simulink model "hydraulicsystem"  (R2020b)
settings: Solver=VariableStepAuto  StartTime=0.0  StopTime=80  FixedStep=0.01  RelTol=1e-3
libraries: fl_lib x15, sh_lib x7, nesl_utility x6, simulink x3, dspstat3 x1, sdl_lib x1
settings Model: EnablePacing=on  PacingRate=2  Creator=mateu  LastModifiedBy=mateu
settings SolverCC: ZeroCrossControl=EnableAll  ZeroCrossAlgorithm=Adaptive  AlgebraicLoopSolver=LineSearch
settings DebuggingCC: IgnoredZcDiagnostic=none
settings SimscapeCC: GlobalZcOffDiagnosticOptions=error  SimscapeLogOpenViewer=on  SimscapeLogLimitData=off

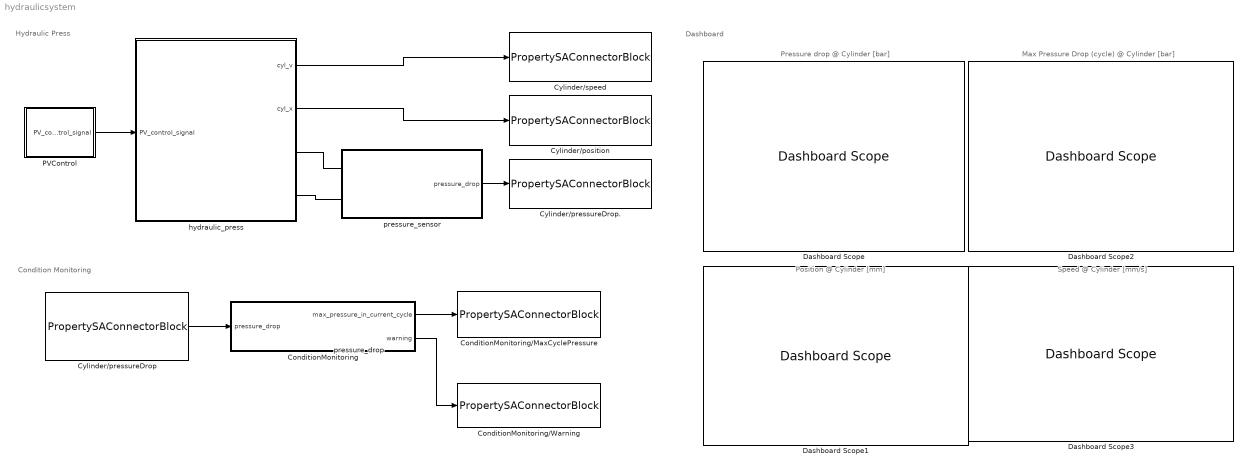
== system hydraulicsystem ==
  note: Dashboard
  note: Hydraulic Press
  note: Condition Monitoring
  note: Pressure drop @ Cylinder [bar]
  note: Max Pressure Drop (cycle) @ Cylinder [bar]
  note: Position @ Cylinder [mm]
  note: Speed @ Cylinder [mm/s]
  pressure_drop : Inport
  ConditionMonitoring : Subsystem
  ConditionMonitoring/MaxCyclePressure : S-Function  FunctionName=PropertySAConnectorBlock  Parameters=bm, sr, regUrlStr, aasUrlStr, aasId, smId, seId  SFunctionDeploymentMode=off  EnableBusSupport=off  mask{bmStr=Real-time, conMethod=via RegistryServer, aasUrlStr_=http://localhost:4001/aasServer/shells/https%3A%2F%2Fexample.com%2Fids%2Faas%2F6001_2130_8022_6165/aas, regUrlStr=http://localhost:8082/registry/api/v1/registry, sr=0.1, aasId=HydraulicPress, smId=ConditionMonitoring, seId=maxCyclePressure, bm=1, aasUrlStr=}
      mask prompts: bmStr "Operation Mode"; conMethod "Connection Method"; aasUrlStr_ "AAS Url"; regUrlStr "Registry URL"; sr "Sample Rate"; aasId "AAS Id"; smId "Submodel IdShort"; seId "Property IdShort"
      mask TypeOptions bmStr: Snapshot | Real-time
      mask Callback bmStr:
      | bmStr = get_param(gcb,'bmStr');
      | vis = get_param(gcb,'MaskVisibilities');
      | 
      | switch bmStr
      |     case 'Snapshot'
      |         set_param(gcb, 'bm', "0");
      |         vis(5) = {'off'};
      |         set_param(gcb, 'MaskVisibilities', vis);
      |     case 'Real-time'
      |         set_param(gcb, 'bm',  "1");
      |         vis(5) = {'on'};
      |         set_param(gcb, 'MaskVisibilities', vis);
      | end
      mask TypeOptions conMethod: via RegistryServer | via AAS URL
      mask Callback conMethod:
      | conMethod = get_param(gcb,'conMethod');
      | aasUrlStr = get_param(gcb,'aasUrlStr_');
      | vis = get_param(gcb,'MaskVisibilities');
      | 
      | switch conMethod
      |     case 'via RegistryServer'
      |         vis(3) = {'off'};
      |         vis(4) = {'on'};
      |         set_param(gcb, 'MaskVisibilities', vis);
      |         set_param(gcb, 'aasUrlStr', '');
      |     case 'via AAS URL'
      |         vis(3) = {'on'};
      |         vis(4) = {'off'};
      |         set_param(gcb, 'MaskVisibilities', vis);
      |         set_param(gcb, 'aasUrlStr', aasUrlStr);
      | end
      mask Callback aasUrlStr_:
      | conMethod = get_param(gcb,'conMethod');
      | aasUrlStr = get_param(gcb,'aasUrlStr_');
      | switch conMethod
      |     case 'via AAS URL'
      |         set_param(gcb, 'aasUrlStr', aasUrlStr);
      | end
      mask DialogControl DescGroupVar Prompt: Standalone Property Block
      mask DialogControl DescTextVar Prompt: This block connects to a SubmodelElement running in an AAS Server. Data sent to the block's input updates the value of the SubmodelElement, whereas its current value is sent to the block's output. This process can be executed in two operation modes: Snapshot mode, wherein the input routine is executed at the beginining and the output routine at the end of the simulation; Real-time mode, by which is assumed that the wall clock is the same as the simulation clock and the input/output routines are executed in the specified sample rate.
      mask Display:
      | bm = get_param(gcb,'bm')
      | sr = get_param(gcb,'sr')
      | aas = replace(get_param(gcb,'aasId'),"_","\_");
      | sm = replace(get_param(gcb,'smId'),"_","\_");
      | se = replace(get_param(gcb,'seId'),"_","\_");
      | 
      | pos = get_param(gcb, 'Position');
      | w = pos(3) - pos(1);
      | h = pos(4) - pos(2);
      | 
      | full = sm  + "/" + se
      | text(5,20, "{\bf\fontsize{7}"+aas+"}", 'texmode','on')
      | text(5,10, "{\bf\fontsize{6}"+full+"}", 'texmode','on')
      | image('basyx.png', [w-15,h-20,10,15]);
      | 
      | if bm=="1"
      |     port_label('output', 1,"{\bf\fontsize{6}sr="+sr+"s}", 'texmode','on')
      | end
  ConditionMonitoring/Warning : S-Function  FunctionName=PropertySAConnectorBlock  Parameters=bm, sr, regUrlStr, aasUrlStr, aasId, smId, seId  SFunctionDeploymentMode=off  EnableBusSupport=off  mask{bmStr=Real-time, conMethod=via RegistryServer, aasUrlStr_=http://localhost:4001/aasServer/shells/https%3A%2F%2Fexample.com%2Fids%2Faas%2F6001_2130_8022_6165/aas, regUrlStr=http://localhost:8082/registry/api/v1/registry, sr=0.1, aasId=HydraulicPress, smId=ConditionMonitoring, seId=warning, bm=1, aasUrlStr=}
      mask prompts: bmStr "Operation Mode"; conMethod "Connection Method"; aasUrlStr_ "AAS Url"; regUrlStr "Registry URL"; sr "Sample Rate"; aasId "AAS Id"; smId "Submodel IdShort"; seId "Property IdShort"
      mask TypeOptions bmStr: Snapshot | Real-time
      mask Callback bmStr:
      | bmStr = get_param(gcb,'bmStr');
      | vis = get_param(gcb,'MaskVisibilities');
      | 
      | switch bmStr
      |     case 'Snapshot'
      |         set_param(gcb, 'bm', "0");
      |         vis(5) = {'off'};
      |         set_param(gcb, 'MaskVisibilities', vis);
      |     case 'Real-time'
      |         set_param(gcb, 'bm',  "1");
      |         vis(5) = {'on'};
      |         set_param(gcb, 'MaskVisibilities', vis);
      | end
      mask TypeOptions conMethod: via RegistryServer | via AAS URL
      mask Callback conMethod:
      | conMethod = get_param(gcb,'conMethod');
      | aasUrlStr = get_param(gcb,'aasUrlStr_');
      | vis = get_param(gcb,'MaskVisibilities');
      | 
      | switch conMethod
      |     case 'via RegistryServer'
      |         vis(3) = {'off'};
      |         vis(4) = {'on'};
      |         set_param(gcb, 'MaskVisibilities', vis);
      |         set_param(gcb, 'aasUrlStr', '');
      |     case 'via AAS URL'
      |         vis(3) = {'on'};
      |         vis(4) = {'off'};
      |         set_param(gcb, 'MaskVisibilities', vis);
      |         set_param(gcb, 'aasUrlStr', aasUrlStr);
      | end
      mask Callback aasUrlStr_:
      | conMethod = get_param(gcb,'conMethod');
      | aasUrlStr = get_param(gcb,'aasUrlStr_');
      | switch conMethod
      |     case 'via AAS URL'
      |         set_param(gcb, 'aasUrlStr', aasUrlStr);
      | end
      mask DialogControl DescGroupVar Prompt: Standalone Property Block
      mask DialogControl DescTextVar Prompt: This block connects to a SubmodelElement running in an AAS Server. Data sent to the block's input updates the value of the SubmodelElement, whereas its current value is sent to the block's output. This process can be executed in two operation modes: Snapshot mode, wherein the input routine is executed at the beginining and the output routine at the end of the simulation; Real-time mode, by which is assumed that the wall clock is the same as the simulation clock and the input/output routines are executed in the specified sample rate.
      mask Display:
      | bm = get_param(gcb,'bm')
      | sr = get_param(gcb,'sr')
      | aas = replace(get_param(gcb,'aasId'),"_","\_");
      | sm = replace(get_param(gcb,'smId'),"_","\_");
      | se = replace(get_param(gcb,'seId'),"_","\_");
      | 
      | pos = get_param(gcb, 'Position');
      | w = pos(3) - pos(1);
      | h = pos(4) - pos(2);
      | 
      | full = sm  + "/" + se
      | text(5,20, "{\bf\fontsize{7}"+aas+"}", 'texmode','on')
      | text(5,10, "{\bf\fontsize{6}"+full+"}", 'texmode','on')
      | image('basyx.png', [w-15,h-20,10,15]);
      | 
      | if bm=="1"
      |     port_label('output', 1,"{\bf\fontsize{6}sr="+sr+"s}", 'texmode','on')
      | end
  Cylinder/position : S-Function  FunctionName=PropertySAConnectorBlock  Parameters=bm, sr, regUrlStr, aasUrlStr, aasId, smId, seId  SFunctionDeploymentMode=off  EnableBusSupport=off  mask{bmStr=Real-time, conMethod=via RegistryServer, aasUrlStr_=http://localhost:4001/aasServer/shells/https%3A%2F%2Fexample.com%2Fids%2Faas%2F6001_2130_8022_6165/aas, regUrlStr=http://localhost:8082/registry/api/v1/registry, sr=0.1, aasId=HydraulicPress, smId=Cylinder, seId=position, bm=1, aasUrlStr=}
      mask prompts: bmStr "Operation Mode"; conMethod "Connection Method"; aasUrlStr_ "AAS Url"; regUrlStr "Registry URL"; sr "Sample Rate"; aasId "AAS Id"; smId "Submodel IdShort"; seId "Property IdShort"
      mask TypeOptions bmStr: Snapshot | Real-time
      mask Callback bmStr:
      | bmStr = get_param(gcb,'bmStr');
      | vis = get_param(gcb,'MaskVisibilities');
      | 
      | switch bmStr
      |     case 'Snapshot'
      |         set_param(gcb, 'bm', "0");
      |         vis(5) = {'off'};
      |         set_param(gcb, 'MaskVisibilities', vis);
      |     case 'Real-time'
      |         set_param(gcb, 'bm',  "1");
      |         vis(5) = {'on'};
      |         set_param(gcb, 'MaskVisibilities', vis);
      | end
      mask TypeOptions conMethod: via RegistryServer | via AAS URL
      mask Callback conMethod:
      | conMethod = get_param(gcb,'conMethod');
      | aasUrlStr = get_param(gcb,'aasUrlStr_');
      | vis = get_param(gcb,'MaskVisibilities');
      | 
      | switch conMethod
      |     case 'via RegistryServer'
      |         vis(3) = {'off'};
      |         vis(4) = {'on'};
      |         set_param(gcb, 'MaskVisibilities', vis);
      |         set_param(gcb, 'aasUrlStr', '');
      |     case 'via AAS URL'
      |         vis(3) = {'on'};
      |         vis(4) = {'off'};
      |         set_param(gcb, 'MaskVisibilities', vis);
      |         set_param(gcb, 'aasUrlStr', aasUrlStr);
      | end
      mask Callback aasUrlStr_:
      | conMethod = get_param(gcb,'conMethod');
      | aasUrlStr = get_param(gcb,'aasUrlStr_');
      | switch conMethod
      |     case 'via AAS URL'
      |         set_param(gcb, 'aasUrlStr', aasUrlStr);
      | end
      mask DialogControl DescGroupVar Prompt: Standalone Property Block
      mask DialogControl DescTextVar Prompt: This block connects to a SubmodelElement running in an AAS Server. Data sent to the block's input updates the value of the SubmodelElement, whereas its current value is sent to the block's output. This process can be executed in two operation modes: Snapshot mode, wherein the input routine is executed at the beginining and the output routine at the end of the simulation; Real-time mode, by which is assumed that the wall clock is the same as the simulation clock and the input/output routines are executed in the specified sample rate.
      mask Display:
      | bm = get_param(gcb,'bm')
      | sr = get_param(gcb,'sr')
      | aas = replace(get_param(gcb,'aasId'),"_","\_");
      | sm = replace(get_param(gcb,'smId'),"_","\_");
      | se = replace(get_param(gcb,'seId'),"_","\_");
      | 
      | pos = get_param(gcb, 'Position');
      | w = pos(3) - pos(1);
      | h = pos(4) - pos(2);
      | 
      | full = sm  + "/" + se
      | text(5,20, "{\bf\fontsize{7}"+aas+"}", 'texmode','on')
      | text(5,10, "{\bf\fontsize{6}"+full+"}", 'texmode','on')
      | image('basyx.png', [w-15,h-20,10,15]);
      | 
      | if bm=="1"
      |     port_label('output', 1,"{\bf\fontsize{6}sr="+sr+"s}", 'texmode','on')
      | end
  Cylinder/pressureDrop : S-Function  FunctionName=PropertySAConnectorBlock  Parameters=bm, sr, regUrlStr, aasUrlStr, aasId, smId, seId  SFunctionDeploymentMode=off  EnableBusSupport=off  mask{bmStr=Real-time, conMethod=via RegistryServer, aasUrlStr_=http://localhost:4001/aasServer/shells/https%3A%2F%2Fexample.com%2Fids%2Faas%2F6001_2130_8022_6165/aas, regUrlStr=http://localhost:8082/registry/api/v1/registry, sr=0.1, aasId=HydraulicPress, smId=Cylinder, seId=pressureDrop, bm=1, aasUrlStr=}
      mask prompts: bmStr "Operation Mode"; conMethod "Connection Method"; aasUrlStr_ "AAS Url"; regUrlStr "Registry URL"; sr "Sample Rate"; aasId "AAS Id"; smId "Submodel IdShort"; seId "Property IdShort"
      mask TypeOptions bmStr: Snapshot | Real-time
      mask Callback bmStr:
      | bmStr = get_param(gcb,'bmStr');
      | vis = get_param(gcb,'MaskVisibilities');
      | 
      | switch bmStr
      |     case 'Snapshot'
      |         set_param(gcb, 'bm', "0");
      |         vis(5) = {'off'};
      |         set_param(gcb, 'MaskVisibilities', vis);
      |     case 'Real-time'
      |         set_param(gcb, 'bm',  "1");
      |         vis(5) = {'on'};
      |         set_param(gcb, 'MaskVisibilities', vis);
      | end
      mask TypeOptions conMethod: via RegistryServer | via AAS URL
      mask Callback conMethod:
      | conMethod = get_param(gcb,'conMethod');
      | aasUrlStr = get_param(gcb,'aasUrlStr_');
      | vis = get_param(gcb,'MaskVisibilities');
      | 
      | switch conMethod
      |     case 'via RegistryServer'
      |         vis(3) = {'off'};
      |         vis(4) = {'on'};
      |         set_param(gcb, 'MaskVisibilities', vis);
      |         set_param(gcb, 'aasUrlStr', '');
      |     case 'via AAS URL'
      |         vis(3) = {'on'};
      |         vis(4) = {'off'};
      |         set_param(gcb, 'MaskVisibilities', vis);
      |         set_param(gcb, 'aasUrlStr', aasUrlStr);
      | end
      mask Callback aasUrlStr_:
      | conMethod = get_param(gcb,'conMethod');
      | aasUrlStr = get_param(gcb,'aasUrlStr_');
      | switch conMethod
      |     case 'via AAS URL'
      |         set_param(gcb, 'aasUrlStr', aasUrlStr);
      | end
      mask DialogControl DescGroupVar Prompt: Standalone Property Block
      mask DialogControl DescTextVar Prompt: This block connects to a SubmodelElement running in an AAS Server. Data sent to the block's input updates the value of the SubmodelElement, whereas its current value is sent to the block's output. This process can be executed in two operation modes: Snapshot mode, wherein the input routine is executed at the beginining and the output routine at the end of the simulation; Real-time mode, by which is assumed that the wall clock is the same as the simulation clock and the input/output routines are executed in the specified sample rate.
      mask Display:
      | bm = get_param(gcb,'bm')
      | sr = get_param(gcb,'sr')
      | aas = replace(get_param(gcb,'aasId'),"_","\_");
      | sm = replace(get_param(gcb,'smId'),"_","\_");
      | se = replace(get_param(gcb,'seId'),"_","\_");
      | 
      | pos = get_param(gcb, 'Position');
      | w = pos(3) - pos(1);
      | h = pos(4) - pos(2);
      | 
      | full = sm  + "/" + se
      | text(5,20, "{\bf\fontsize{7}"+aas+"}", 'texmode','on')
      | text(5,10, "{\bf\fontsize{6}"+full+"}", 'texmode','on')
      | image('basyx.png', [w-15,h-20,10,15]);
      | 
      | if bm=="1"
      |     port_label('output', 1,"{\bf\fontsize{6}sr="+sr+"s}", 'texmode','on')
      | end
  Cylinder/pressureDrop. : S-Function  FunctionName=PropertySAConnectorBlock  Parameters=bm, sr, regUrlStr, aasUrlStr, aasId, smId, seId  SFunctionDeploymentMode=off  EnableBusSupport=off  mask{bmStr=Real-time, conMethod=via RegistryServer, aasUrlStr_=http://localhost:4001/aasServer/shells/https%3A%2F%2Fexample.com%2Fids%2Faas%2F6001_2130_8022_6165/aas, regUrlStr=http://localhost:8082/registry/api/v1/registry, sr=0.05, aasId=HydraulicPress, smId=Cylinder, seId=pressureDrop, bm=1, aasUrlStr=}
      mask prompts: bmStr "Operation Mode"; conMethod "Connection Method"; aasUrlStr_ "AAS Url"; regUrlStr "Registry URL"; sr "Sample Rate"; aasId "AAS Id"; smId "Submodel IdShort"; seId "Property IdShort"
      mask TypeOptions bmStr: Snapshot | Real-time
      mask Callback bmStr:
      | bmStr = get_param(gcb,'bmStr');
      | vis = get_param(gcb,'MaskVisibilities');
      | 
      | switch bmStr
      |     case 'Snapshot'
      |         set_param(gcb, 'bm', "0");
      |         vis(5) = {'off'};
      |         set_param(gcb, 'MaskVisibilities', vis);
      |     case 'Real-time'
      |         set_param(gcb, 'bm',  "1");
      |         vis(5) = {'on'};
      |         set_param(gcb, 'MaskVisibilities', vis);
      | end
      mask TypeOptions conMethod: via RegistryServer | via AAS URL
      mask Callback conMethod:
      | conMethod = get_param(gcb,'conMethod');
      | aasUrlStr = get_param(gcb,'aasUrlStr_');
      | vis = get_param(gcb,'MaskVisibilities');
      | 
      | switch conMethod
      |     case 'via RegistryServer'
      |         vis(3) = {'off'};
      |         vis(4) = {'on'};
      |         set_param(gcb, 'MaskVisibilities', vis);
      |         set_param(gcb, 'aasUrlStr', '');
      |     case 'via AAS URL'
      |         vis(3) = {'on'};
      |         vis(4) = {'off'};
      |         set_param(gcb, 'MaskVisibilities', vis);
      |         set_param(gcb, 'aasUrlStr', aasUrlStr);
      | end
      mask Callback aasUrlStr_:
      | conMethod = get_param(gcb,'conMethod');
      | aasUrlStr = get_param(gcb,'aasUrlStr_');
      | switch conMethod
      |     case 'via AAS URL'
      |         set_param(gcb, 'aasUrlStr', aasUrlStr);
      | end
      mask DialogControl DescGroupVar Prompt: Standalone Property Block
      mask DialogControl DescTextVar Prompt: This block connects to a SubmodelElement running in an AAS Server. Data sent to the block's input updates the value of the SubmodelElement, whereas its current value is sent to the block's output. This process can be executed in two operation modes: Snapshot mode, wherein the input routine is executed at the beginining and the output routine at the end of the simulation; Real-time mode, by which is assumed that the wall clock is the same as the simulation clock and the input/output routines are executed in the specified sample rate.
      mask Display:
      | bm = get_param(gcb,'bm')
      | sr = get_param(gcb,'sr')
      | aas = replace(get_param(gcb,'aasId'),"_","\_");
      | sm = replace(get_param(gcb,'smId'),"_","\_");
      | se = replace(get_param(gcb,'seId'),"_","\_");
      | 
      | pos = get_param(gcb, 'Position');
      | w = pos(3) - pos(1);
      | h = pos(4) - pos(2);
      | 
      | full = sm  + "/" + se
      | text(5,20, "{\bf\fontsize{7}"+aas+"}", 'texmode','on')
      | text(5,10, "{\bf\fontsize{6}"+full+"}", 'texmode','on')
      | image('basyx.png', [w-15,h-20,10,15]);
      | 
      | if bm=="1"
      |     port_label('output', 1,"{\bf\fontsize{6}sr="+sr+"s}", 'texmode','on')
      | end
  Cylinder/speed : S-Function  FunctionName=PropertySAConnectorBlock  Parameters=bm, sr, regUrlStr, aasUrlStr, aasId, smId, seId  SFunctionDeploymentMode=off  EnableBusSupport=off  mask{bmStr=Real-time, conMethod=via RegistryServer, aasUrlStr_=http://localhost:4001/aasServer/shells/https%3A%2F%2Fexample.com%2Fids%2Faas%2F6001_2130_8022_6165/aas, regUrlStr=http://localhost:8082/registry/api/v1/registry, sr=0.1, aasId=HydraulicPress, smId=Cylinder, seId=speed, bm=1, aasUrlStr=}
      mask prompts: bmStr "Operation Mode"; conMethod "Connection Method"; aasUrlStr_ "AAS Url"; regUrlStr "Registry URL"; sr "Sample Rate"; aasId "AAS Id"; smId "Submodel IdShort"; seId "Property IdShort"
      mask TypeOptions bmStr: Snapshot | Real-time
      mask Callback bmStr:
      | bmStr = get_param(gcb,'bmStr');
      | vis = get_param(gcb,'MaskVisibilities');
      | 
      | switch bmStr
      |     case 'Snapshot'
      |         set_param(gcb, 'bm', "0");
      |         vis(5) = {'off'};
      |         set_param(gcb, 'MaskVisibilities', vis);
      |     case 'Real-time'
      |         set_param(gcb, 'bm',  "1");
      |         vis(5) = {'on'};
      |         set_param(gcb, 'MaskVisibilities', vis);
      | end
      mask TypeOptions conMethod: via RegistryServer | via AAS URL
      mask Callback conMethod:
      | conMethod = get_param(gcb,'conMethod');
      | aasUrlStr = get_param(gcb,'aasUrlStr_');
      | vis = get_param(gcb,'MaskVisibilities');
      | 
      | switch conMethod
      |     case 'via RegistryServer'
      |         vis(3) = {'off'};
      |         vis(4) = {'on'};
      |         set_param(gcb, 'MaskVisibilities', vis);
      |         set_param(gcb, 'aasUrlStr', '');
      |     case 'via AAS URL'
      |         vis(3) = {'on'};
      |         vis(4) = {'off'};
      |         set_param(gcb, 'MaskVisibilities', vis);
      |         set_param(gcb, 'aasUrlStr', aasUrlStr);
      | end
      mask Callback aasUrlStr_:
      | conMethod = get_param(gcb,'conMethod');
      | aasUrlStr = get_param(gcb,'aasUrlStr_');
      | switch conMethod
      |     case 'via AAS URL'
      |         set_param(gcb, 'aasUrlStr', aasUrlStr);
      | end
      mask DialogControl DescGroupVar Prompt: Standalone Property Block
      mask DialogControl DescTextVar Prompt: This block connects to a SubmodelElement running in an AAS Server. Data sent to the block's input updates the value of the SubmodelElement, whereas its current value is sent to the block's output. This process can be executed in two operation modes: Snapshot mode, wherein the input routine is executed at the beginining and the output routine at the end of the simulation; Real-time mode, by which is assumed that the wall clock is the same as the simulation clock and the input/output routines are executed in the specified sample rate.
      mask Display:
      | bm = get_param(gcb,'bm')
      | sr = get_param(gcb,'sr')
      | aas = replace(get_param(gcb,'aasId'),"_","\_");
      | sm = replace(get_param(gcb,'smId'),"_","\_");
      | se = replace(get_param(gcb,'seId'),"_","\_");
      | 
      | pos = get_param(gcb, 'Position');
      | w = pos(3) - pos(1);
      | h = pos(4) - pos(2);
      | 
      | full = sm  + "/" + se
      | text(5,20, "{\bf\fontsize{7}"+aas+"}", 'texmode','on')
      | text(5,10, "{\bf\fontsize{6}"+full+"}", 'texmode','on')
      | image('basyx.png', [w-15,h-20,10,15]);
      | 
      | if bm=="1"
      |     port_label('output', 1,"{\bf\fontsize{6}sr="+sr+"s}", 'texmode','on')
      | end
  Dashboard Scope : DashboardScope  TimeSpan=20  Ymin=-200  Ymax=205  LegendPosition=Hide  ScaleAtStop=off
  Dashboard Scope1 : DashboardScope  TimeSpan=20  Ymin=-305  Ymax=305  LegendPosition=Hide  ScaleAtStop=off
  Dashboard Scope2 : DashboardScope  ShowInitialText=off  Ymin=199  Ymax=201  LegendPosition=Hide  ScaleAtStop=off
  Dashboard Scope3 : DashboardScope  TimeSpan=20  Ymin=-100  Ymax=100  LegendPosition=Hide  ScaleAtStop=off
  PVControl : Subsystem
  hydraulic_press : Subsystem
  pressure_sensor : Subsystem
  wires:
  Cylinder/pressureDrop/1 -> ConditionMonitoring/1(pressure_drop)
  PVControl/1(PV_control_signal) -> hydraulic_press/1(PV_control_signal)
  pressure_sensor/1(pressure_drop) -> Cylinder/pressureDrop./1
  hydraulic_press/2(cyl_x) -> Cylinder/position/1
  hydraulic_press/1(cyl_v) -> Cylinder/speed/1
  ConditionMonitoring/1(max_pressure_in_current_cycle) -> ConditionMonitoring/MaxCyclePressure/1
  ConditionMonitoring/2(warning) -> ConditionMonitoring/Warning/1
  connections:
  hydraulic_press/RConn2 -- pressure_sensor/LConn2
  pressure_sensor/LConn1 -- hydraulic_press/RConn1

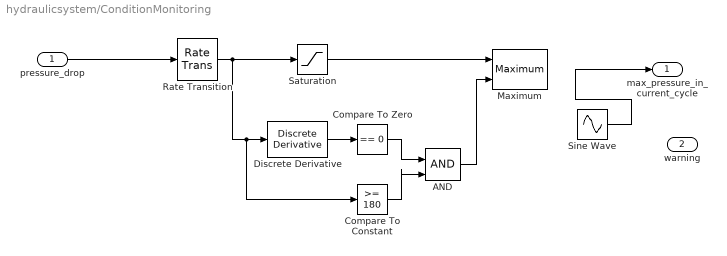
== system hydraulicsystem/ConditionMonitoring ==
  pressure_drop : Inport
  AND : Logic  IconShape=distinctive  AllPortsSameDT=off  OutDataTypeStr=boolean
  Compare To Constant : simulink/Logic and Bit Operations/Compare To Constant  relop=>=  const=180  OutDataTypeStr=boolean
  Compare To Zero : simulink/Logic and Bit Operations/Compare To Zero  relop===  OutDataTypeStr=boolean
  Discrete Derivative : simulink/Discrete/Discrete Derivative  gainval=1.0  ICPrevScaledInput=0.0  OutMin=[]  OutMax=[]  OutDataType=fixdt(1, 16)  OutScaling=2^-10  DoSatur=off
  Maximum : dspstat3/Maximum  operation=maximum  fcn=Running  indexBase=One  operateOver=Entire input  Dimension=100  InputProcessing=Columns as channels (frame based)  reset=Non-zero sample  roiEnable=off  roiType=Rectangles  roiPortion=Entire ROI  roiOutput=Individual statistics for each ROI  roiFlag=off  roundingMode=Floor  overflowMode=off  accumDataTypeStr=Inherit: Same as product output  accumLastDataTypeStr=Inherit: Same as product output
  Rate Transition : RateTransition  OutPortSampleTime=.1
  Saturation : Saturate  UpperLimit=300  LowerLimit=100
  Sine Wave : Sin  Amplitude=200  Frequency=0.0005  Phase=pi/2  SampleTime=15
  max_pressure_in_current_cycle : Outport
  warning : Outport  Port=2
  wires:
  Rate Transition/1 -> Compare To Constant/1, Discrete Derivative/1, Saturation/1
  Compare To Zero/1 -> AND/1
  Compare To Constant/1 -> AND/2
  Discrete Derivative/1 -> Compare To Zero/1
  Saturation/1 -> Maximum/1
  AND/1 -> Maximum/2
  Sine Wave/1 -> max_pressure_in_current_cycle/1
  pressure_drop/1 -> Rate Transition/1

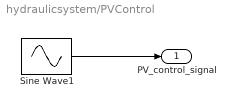
== system hydraulicsystem/PVControl ==
  Sine Wave1 : Sin  Amplitude=0.003  Frequency=2*3.14/(10)/2  SampleTime=0.1
  PV_control_signal : Outport
  wires:
  Sine Wave1/1 -> PV_control_signal/1

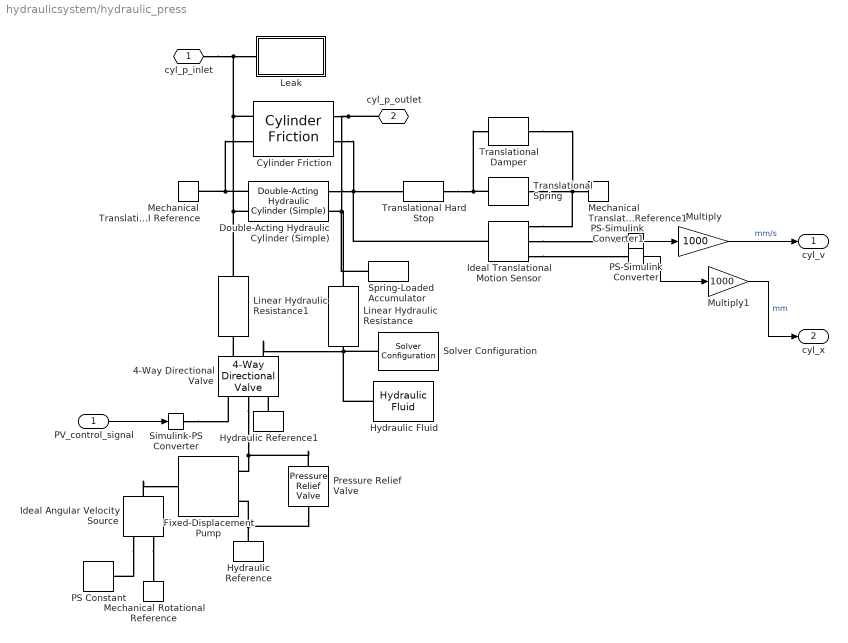
== system hydraulicsystem/hydraulic_press ==
  PV_control_signal : Inport
  4-Way Directional Valve : sh_lib/Valves/Directional Valves/4-Way Directional Valve  area_spec=sh.valves.directional_valves.enum.area_spec.identical  x_0_P_A=0 m  x_0_P_B=0 m  x_0_A_T=0 m  x_0_B_T=0 m  mdl_type_identical=sh.valves.directional_valves.enum.mdl_type.linear  mdl_type_different=sh.valves.directional_valves.enum.mdl_type.linear  opening_max=0.005 m  area_max=0.5e-4 m^2  opening_max_P_A=0.005 m  area_max_P_A=0.5e-4 m^2  opening_max_P_B=0.005 m  area_max_P_B=0.5e-4 m^2  opening_max_A_T=0.005 m  area_max_A_T=0.5e-4 m^2  opening_max_B_T=0.005 m  area_max_B_T=0.5e-4 m^2  opening_area_tab=[-.002, 0, .002, .005, .015] m  area_tab=[1e-09, 2.0352e-07, 4.0736e-05, .00011438, .00034356] m^2  opening_flow_rate_tab=[-.002, 0, .002, .005, .015] m  pressure_tab=[-10000000, -5000000, -2000000, 2000000, 5000000, 10000000] Pa  flow_rate_tab=[-1e-07, -7.0711e-08, -4.4721e-08, 4.4721e-08, 7.0711e-08, 1e-07; -2.0352e-05, -1.4391e-05, -9.1017e-06, 9.1017e-06, 1.4391e-05, 2.0352e-05; -.0040736, -.0028805, -.0018218, .0018218, .0028805, .0040736; -.011438, -.0080879, -.0051152, .0051152, .0080879, .011438; -.034356, -.024293, -.015364, .015364, .024293, .034356] m^3/s  opening_area_tab_P_A=[-.002, 0, .002, .005, .015] m  area_tab_P_A=[1e-09, 2.0352e-07, 4.0736e-05, .00011438, .00034356] m^2  opening_flow_rate_tab_P_A=[-.002, 0, .002, .005, .015] m  pressure_tab_P_A=[-10000000, -5000000, -2000000, 2000000, 5000000, 10000000] Pa  flow_rate_tab_P_A=[-1e-07, -7.0711e-08, -4.4721e-08, 4.4721e-08, 7.0711e-08, 1e-07; -2.0352e-05, -1.4391e-05, -9.1017e-06, 9.1017e-06, 1.4391e-05, 2.0352e-05; -.0040736, -.0028805, -.0018218, .0018218, .0028805, .0040736; -.011438, -.0080879, -.0051152, .0051152, .0080879, .011438; -.034356, -.024293, -.015364, .015364, .024293, .034356] m^3/s  opening_area_tab_P_B=[-.002, 0, .002, .005, .015] m  area_tab_P_B=[1e-09, 2.0352e-07, 4.0736e-05, .00011438, .00034356] m^2  opening_flow_rate_tab_P_B=[-.002, 0, .002, .005, .015] m  pressure_tab_P_B=[-10000000, -5000000, -2000000, 2000000, 5000000, 10000000] Pa  flow_rate_tab_P_B=[-1e-07, -7.0711e-08, -4.4721e-08, 4.4721e-08, 7.0711e-08, 1e-07; -2.0352e-05, -1.4391e-05, -9.1017e-06, 9.1017e-06, 1.4391e-05, 2.0352e-05; -.0040736, -.0028805, -.0018218, .0018218, .0028805, .0040736; -.011438, -.0080879, -.0051152, .0051152, .0080879, .011438; -.034356, -.024293, -.015364, .015364, .024293, .034356] m^3/s  opening_area_tab_A_T=[-.002, 0, .002, .005, .015] m  area_tab_A_T=[1e-09, 2.0352e-07, 4.0736e-05, .00011438, .00034356] m^2  opening_flow_rate_tab_A_T=[-.002, 0, .002, .005, .015] m  pressure_tab_A_T=[-10000000, -5000000, -2000000, 2000000, 5000000, 10000000] Pa  flow_rate_tab_A_T=[-1e-07, -7.0711e-08, -4.4721e-08, 4.4721e-08, 7.0711e-08, 1e-07; -2.0352e-05, -1.4391e-05, -9.1017e-06, 9.1017e-06, 1.4391e-05, 2.0352e-05; -.0040736, -.0028805, -.0018218, .0018218, .0028805, .0040736; -.011438, -.0080879, -.0051152, .0051152, .0080879, .011438; -.034356, -.024293, -.015364, .015364, .024293, .034356] m^3/s  opening_area_tab_B_T=[-.002, 0, .002, .005, .015] m  area_tab_B_T=[1e-09, 2.0352e-07, 4.0736e-05, .00011438, .00034356] m^2  opening_flow_rate_tab_B_T=[-.002, 0, .002, .005, .015] m  pressure_tab_B_T=[-10000000, -5000000, -2000000, 2000000, 5000000, 10000000] Pa  flow_rate_tab_B_T=[-1e-07, -7.0711e-08, -4.4721e-08, 4.4721e-08, 7.0711e-08, 1e-07; -2.0352e-05, -1.4391e-05, -9.1017e-06, 9.1017e-06, 1.4391e-05, 2.0352e-05; -.0040736, -.0028805, -.0018218, .0018218, .0028805, .0040736; -.011438, -.0080879, -.0051152, .0051152, .0080879, .011438; -.034356, -.024293, -.015364, .015364, .024293, .034356] m^3/s  interp_method_identical=sh.valves.directional_valves.enum.interp_method.linear  interp_method_different=sh.valves.directional_valves.enum.interp_method.linear  extrap_method_identical=sh.valves.directional_valves.enum.extrap_method.linear  extrap_method_different=sh.valves.directional_valves.enum.extrap_method.linear  A_leak=1e-12 m^2  C_d=0.7  lam_spec=sh.valves.directional_valves.enum.lam_spec.pressure_ratio  B_lam=0.999  Re_cr=12
      settings: SourceProductBaseCode=SH  InternalSimscapePortConfiguration="{\"Bottom\":[],\"Left\":[{\"id\":\"A\",\"label\":\"A\",\"type\":\"foundation.hydraulic.hydraulic\"},{\"id\":\"B\",\"label\":\"B\",\"type\":\"foundation.hydraulic.hydraulic\"}],\"Right\":[{\"id\":\"S\",\"label\":\"S\",\"type\":\"input\"},{\"id\":\"P\",\"label\":\"P\",\"type\":\"foundation.hydraulic.hydraulic\"},{\"id\":\"T\",\"label\":\"T\",\"type\":\"foundation.hydraulic.hydraulic\"}],\"Top\":[]}"
  Cylinder Friction : sh_lib/Hydraulic Cylinders/Cylinder Friction  frc_preload=500 N  fr_coef=1e-6 N/Pa  frc_brkwy_coef=1  visc_coef=100 N/(m/s)  trans_coef=10 s/m  vel_thr=1e-4 m/s  flow_rate_A_specify=off  flow_rate_A_priority=None  flow_rate_A=0 m^3/s  flow_rate_A_nominal_specify=off  flow_rate_A_nominal_unit=m^3/s  flow_rate_A_nominal_value=1  flow_rate_B_specify=off  flow_rate_B_priority=None  flow_rate_B=0 m^3/s  flow_rate_B_nominal_specify=off  flow_rate_B_nominal_unit=m^3/s  flow_rate_B_nominal_value=1  friction_force_specify=off  friction_force_priority=None  friction_force=0 N  friction_force_nominal_specify=off  friction_force_nominal_unit=N  friction_force_nominal_value=1  rel_velocity_specify=off  rel_velocity_priority=None  rel_velocity=0 m/s  rel_velocity_nominal_specify=off  rel_velocity_nominal_unit=m/s  rel_velocity_nominal_value=1
      settings: SourceProductBaseCode=SH  InternalSimscapePortConfiguration="{\"Bottom\":[],\"Left\":[{\"id\":\"A\",\"label\":\"A\",\"type\":\"foundation.hydraulic.hydraulic\"},{\"id\":\"C\",\"label\":\"C\",\"type\":\"foundation.mechanical.translational.translational\"}],\"Right\":[{\"id\":\"B\",\"label\":\"B\",\"type\":\"foundation.hydraulic.hydraulic\"},{\"id\":\"R\",\"label\":\"R\",\"type\":\"foundation.mechanical.translational.translational\"}],\"Top\":[]}"
  Double-Acting Hydraulic Cylinder (Simple) : sh_lib/Hydraulic Cylinders/Double-Acting Hydraulic Cylinder (Simple)  area_A=80^2*3.14/4 mm^2  area_B=45^2*3.14/4 mm^2  stroke=300 mm  init_pos=0 m  penetr_coeff=1e12 s*N/m^2  or=1
      settings: SourceProductBaseCode=SH  LogSimulationData=on  InternalSimscapePortConfiguration="{\"Bottom\":[],\"Left\":[{\"id\":\"C\",\"label\":\"C\",\"type\":\"foundation.mechanical.translational.translational\"},{\"id\":\"A\",\"label\":\"A\",\"type\":\"foundation.hydraulic.hydraulic\"}],\"Right\":[{\"id\":\"R\",\"label\":\"R\",\"type\":\"foundation.mechanical.translational.translational\"},{\"id\":\"B\",\"label\":\"B\",\"type\":\"foundation.hydraulic.hydraulic\"}],\"Top\":[]}"
  Fixed-Displacement Pump : sh_lib/Pumps and Motors/Fixed-Displacement Pump  D=12/188 l/rev  loss_spec=1  w_nominal=188 rpm  pr_nominal=100 bar  visc_nominal=18 cSt  dens_nominal=900 kg/m^3  efficiency_vol=0.92  no_load_torque=0.05 N*m  torque_pressure_coeff=0.6e-6 N*m/Pa  p_diff_eff_TLU=[100000, 1000000, 2000000] Pa  omega_eff_TLU=[25, 50, 100, 200, 300, 400] rad/s  vol_eff_TLU=[.816, .908, .954, .977, .981, .984; .325, .663, .831, .916, .925, .946; .137, .568, .78, .892, .893, .91]  mech_eff_TLU=[.996, .996, .996, .996, .996, .996; .988, .989, .989, .989, .989, .99; .981, .981, .982, .982, .983, .984]  p_diff_loss_TLU=[100000, 1000000, 2000000] Pa  omega_loss_TLU=[25, 50, 100, 200, 300, 400] rad/s  vol_loss_TLU=[.023, .023, .023, .023, .0285, .032; .0844, .0842, .0845, .084, .1125, .108; .1079, .108, .11, .108, .1605, .18] * 1e-3 m^3/s  mech_loss_TLU=[.002, .002, .002, .002, .002, .002; .0607, .0556, .0556, .0556, .0556, .0505; .1937, .1937, .1833, .1833, .1729, .1626] N*m  pressure_threshold=1e5 Pa  omega_threshold=10 rad/s  quadrant_check=0  pressure_check=0  min_valid_pressure=0 Pa  vol_eff_min=1e-3  vol_eff_max=1  mech_eff_min=1e-3  mech_eff_max=1
      settings: SourceProductBaseCode=SH  InternalSimscapePortConfiguration="{\"Bottom\":[],\"Left\":[{\"id\":\"S\",\"label\":\"S\",\"type\":\"foundation.mechanical.rotational.rotational\"}],\"Right\":[{\"id\":\"P\",\"label\":\"P\",\"type\":\"foundation.hydraulic.hydraulic\"},{\"id\":\"T\",\"label\":\"T\",\"type\":\"foundation.hydraulic.hydraulic\"}],\"Top\":[]}"
  Hydraulic Fluid : sh_lib/Hydraulic Utilities/Hydraulic Fluid  DataSource=1  SelFluid=1  SysTemp=60  TrapAir=0.005  ViscDerFactor=1  range_error=2
  Hydraulic Reference : fl_lib/Hydraulic/Hydraulic Elements/Hydraulic Reference
  Hydraulic Reference1 : fl_lib/Hydraulic/Hydraulic Elements/Hydraulic Reference
  Ideal Angular Velocity Source : fl_lib/Mechanical/Mechanical Sources/Ideal Angular Velocity Source
  Ideal Translational Motion Sensor : fl_lib/Mechanical/Mechanical Sensors/Ideal Translational Motion Sensor  offset=0 m
  Leak : Subsystem
  Linear Hydraulic Resistance : fl_lib/Hydraulic/Hydraulic Elements/Linear Hydraulic Resistance  resistance=10e9 Pa/(m^3/s)  q_specify=off  q_priority=None  q=0.001 m^3/s  q_nominal_specify=off  q_nominal_unit=m^3/s  q_nominal_value=1  p_specify=off  p_priority=None  p=0 Pa  p_nominal_specify=off  p_nominal_unit=Pa  p_nominal_value=1
      settings: SourceProductBaseCode=SS  InternalSimscapePortConfiguration="{\"Bottom\":[],\"Left\":[{\"id\":\"A\",\"label\":\"A\",\"type\":\"foundation.hydraulic.hydraulic\"}],\"Right\":[{\"id\":\"B\",\"label\":\"B\",\"type\":\"foundation.hydraulic.hydraulic\"}],\"Top\":[]}"
  Linear Hydraulic Resistance1 : fl_lib/Hydraulic/Hydraulic Elements/Linear Hydraulic Resistance  resistance=10e9 Pa/(m^3/s)  q_specify=off  q_priority=None  q=0.001 m^3/s  q_nominal_specify=off  q_nominal_unit=m^3/s  q_nominal_value=1  p_specify=off  p_priority=None  p=0 Pa  p_nominal_specify=off  p_nominal_unit=Pa  p_nominal_value=1
      settings: SourceProductBaseCode=SS  InternalSimscapePortConfiguration="{\"Bottom\":[],\"Left\":[{\"id\":\"A\",\"label\":\"A\",\"type\":\"foundation.hydraulic.hydraulic\"}],\"Right\":[{\"id\":\"B\",\"label\":\"B\",\"type\":\"foundation.hydraulic.hydraulic\"}],\"Top\":[]}"
  Mechanical Rotational Reference : fl_lib/Mechanical/Rotational Elements/Mechanical Rotational Reference
  Mechanical Translational Reference : fl_lib/Mechanical/Translational Elements/Mechanical Translational Reference
  Mechanical Translational Reference1 : fl_lib/Mechanical/Translational Elements/Mechanical Translational Reference
  Multiply : Gain  Gain=1000
  Multiply1 : Gain  Gain=1000
  PS Constant : fl_lib/Physical Signals/Sources/PS Constant  constant=188 rpm
  PS-Simulink Converter : nesl_utility/PS-Simulink Converter  PhysicalDomain=network_engine_domain  SubClassName=ps_output  LeftPortType=input  RightPortType=output  PseudoPeriodic=off  Frequencies=[]  Unit=inherit  AffineConversion=off
  PS-Simulink Converter1 : nesl_utility/PS-Simulink Converter  PhysicalDomain=network_engine_domain  SubClassName=ps_output  LeftPortType=input  RightPortType=output  PseudoPeriodic=off  Frequencies=[]  Unit=inherit  AffineConversion=off
  Pressure Relief Valve : sh_lib/Valves/Pressure Control Valves/Pressure Relief Valve  valve_area_spec=1  p_diff_TLU=[30.15e5 : 15e3 : 31.35e5] Pa  area_TLU=[1 : 1 : 9] .* 1e-5 m^2  area_max=2e-3 m^2  pres_set=200 bar  reg_range=300 bar  C_d=0.7  A_leak=1e-12 m^2  lam_spec=1  B_lam=0.999  Re_cr=12  dynamic=0  tau=0.1 s  area_init=1e-12 m^2
      settings: SourceProductBaseCode=SH  InternalSimscapePortConfiguration="{\"Bottom\":[],\"Left\":[{\"id\":\"A\",\"label\":\"A\",\"type\":\"foundation.hydraulic.hydraulic\"}],\"Right\":[{\"id\":\"B\",\"label\":\"B\",\"type\":\"foundation.hydraulic.hydraulic\"}],\"Top\":[]}"
  Simulink-PS Converter : nesl_utility/Simulink-PS Converter  PhysicalDomain=network_engine_domain  SubClassName=ps_input  LeftPortType=input  RightPortType=output  PseudoPeriodic=off  Frequencies=[]  NoiseDistribution=none  NoiseParameters=[]  Unit=1  AffineConversion=off  FilteringAndDerivatives=provide  SimscapeFilterOrder=1  InputFilterTimeConstant=0.001  UdotUserProvided=0
  Solver Configuration : nesl_utility/Solver Configuration  PhysicalDomain=network_engine_domain  SubClassName=solver  LeftPortType=input  RightPortType=generic  Tones=[]  Harmonics=[]  SimulateNoise=off  Profile=off  UseLocalSampling=off  EnableSwitchedLinearOptims=on  FrequencyDomain=off  UseCCode=off  RelTol=0.001  AbsTol=1e-06  MinStep=1e-09  ToWorkspace=off  RevertToSquareIcSolve=off  NumHomotopyIterations=100  PhasorMode=off  PhasorModeNumHarmonics=1  DoDC=off  ResidualTolerance=1e-09  UseLocalSolver=off  LocalSolverChoice=NE_BACKWARD_EULER_ADVANCER  LocalSolverSampleTime=0.001  DoFixedCost=off  MaxNonlinIter=3  MaxModeIter=2  ComputeImpulses=off  ImpulseIterations=2  LinearAlgebra=auto  EquationFormulation=NE_TIME_EF  DelaysMemoryBudget=1024  AutomaticFiltering=on  FilteringTimeConstant=0.001  PartitionStorageMethod=AS_NEEDED  PartitionMemoryBudget=1024  PartitionMethod=ROBUST
  Spring-Loaded Accumulator : sh_lib/Accumulators/Spring-Loaded Accumulator  capacity=8e-5 m^3  pr_preload=200 bar  pr_max=300 bar  stiff_coeff=1e10 Pa/m^3  penetr_coeff=1e10 s*Pa/m^6  flow_rate_specify=off  flow_rate_priority=High  flow_rate=0.005 m^3/s  flow_rate_nominal_specify=off  flow_rate_nominal_unit=m^3/s  flow_rate_nominal_value=1  fluid_volume_specify=on  fluid_volume_priority=High  fluid_volume=0 m^3  fluid_volume_nominal_specify=off  fluid_volume_nominal_unit=m^3  fluid_volume_nominal_value=1  fluid_pressure_specify=off  fluid_pressure_priority=Low  fluid_pressure=1 bar  fluid_pressure_nominal_specify=off  fluid_pressure_nominal_unit=Pa  fluid_pressure_nominal_value=1
      settings: SourceProductBaseCode=SH  InternalSimscapePortConfiguration="{\"Bottom\":[],\"Left\":[],\"Right\":[{\"id\":\"A\",\"label\":\"A\",\"type\":\"foundation.hydraulic.hydraulic\"}],\"Top\":[]}"
  Translational Damper : sdl_lib/Couplings & Drives/Springs & Dampers/Translational Damper  D=10000 N/(m/s)  enable_faults=0  b_fault=1e6 N/(m/s)  temporal_fault=1  fault_time=5 s  shock_fault=0  acceleration_limit=100 m/s^2  shock_limit=1  report_fault=1
      settings: SourceProductBaseCode=LD  LogSimulationData=on
  Translational Hard Stop : fl_lib/Mechanical/Translational Elements/Translational Hard Stop  upper_bnd=200 mm  lower_bnd=-100 mm  stiff_up=1000 kN/mm  stiff_low=1000 kN/mm  D_up=1000000000 N/(m/s)  D_low=1000000000 N/(m/s)  model=simscape.enum.hardstop.smooth  transition=0.1 mm  v_specify=off  v_priority=None  v=0 m/s  v_nominal_specify=off  v_nominal_unit=m/s  v_nominal_value=1  f_specify=off  f_priority=None  f=0 N  f_nominal_specify=off  f_nominal_unit=N  f_nominal_value=1  x_specify=off  x_priority=High  x=0 m  x_nominal_specify=off  x_nominal_unit=m  x_nominal_value=1
  Translational Spring : fl_lib/Mechanical/Translational Elements/Translational Spring  spr_rate=80/100 kN/mm  v_specify=off  v_priority=None  v=0 m/s  v_nominal_specify=off  v_nominal_unit=m/s  v_nominal_value=1  f_specify=off  f_priority=None  f=0 N  f_nominal_specify=off  f_nominal_unit=N  f_nominal_value=1  x_specify=off  x_priority=High  x=0 m  x_nominal_specify=off  x_nominal_unit=m  x_nominal_value=1
      settings: LogSimulationData=on
  cyl_p_inlet : PMIOPort  Side=Right
  cyl_p_outlet : PMIOPort  Port=2  Side=Right
  cyl_v : Outport
  cyl_x : Outport  Port=2
  wires:
  PV_control_signal/1 -> Simulink-PS Converter/1
  PS-Simulink Converter/1 -> Multiply/1
  Multiply/1 -> cyl_v/1  "mm/s"
  PS-Simulink Converter1/1 -> Multiply1/1
  Multiply1/1 -> cyl_x/1  "mm"
  connections:
  Ideal Angular Velocity Source/RConn1 -- PS Constant/RConn1
  Cylinder Friction/RConn1 -- cyl_p_outlet/RConn1 -- Linear Hydraulic Resistance/RConn1 -- Spring-Loaded Accumulator/RConn1 -- Double-Acting Hydraulic Cylinder (Simple)/RConn2
  Double-Acting Hydraulic Cylinder (Simple)/LConn2 -- Linear Hydraulic Resistance1/RConn1 -- Cylinder Friction/LConn1 -- cyl_p_inlet/RConn1 -- Leak/LConn1
  Ideal Angular Velocity Source/LConn1 -- Fixed-Displacement Pump/LConn1
  Ideal Angular Velocity Source/RConn2 -- Mechanical Rotational Reference/LConn1
  Double-Acting Hydraulic Cylinder (Simple)/RConn1 -- Cylinder Friction/RConn2 -- Ideal Translational Motion Sensor/LConn1 -- Translational Hard Stop/LConn1
  4-Way Directional Valve/LConn2 -- Hydraulic Fluid/RConn1 -- Linear Hydraulic Resistance/LConn1 -- Solver Configuration/RConn1
  Translational Damper/RConn1 -- Translational Spring/RConn1 -- Ideal Translational Motion Sensor/RConn1 -- Mechanical Translational Reference1/LConn1
  Simulink-PS Converter/RConn1 -- 4-Way Directional Valve/RConn1
  Double-Acting Hydraulic Cylinder (Simple)/LConn1 -- Cylinder Friction/LConn2 -- Mechanical Translational Reference/LConn1
  Pressure Relief Valve/LConn1 -- 4-Way Directional Valve/RConn2 -- Fixed-Displacement Pump/RConn1
  Translational Hard Stop/RConn1 -- Translational Spring/LConn1 -- Translational Damper/LConn1
  Hydraulic Reference/LConn1 -- Pressure Relief Valve/RConn1 -- Fixed-Displacement Pump/RConn2
  4-Way Directional Valve/LConn1 -- Linear Hydraulic Resistance1/LConn1
  Hydraulic Reference1/LConn1 -- 4-Way Directional Valve/RConn3
  Ideal Translational Motion Sensor/RConn3 -- PS-Simulink Converter1/LConn1
  Ideal Translational Motion Sensor/RConn2 -- PS-Simulink Converter/LConn1

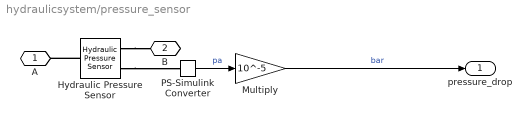
== system hydraulicsystem/pressure_sensor ==
  Hydraulic Pressure Sensor : fl_lib/Hydraulic/Hydraulic Sensors/Hydraulic Pressure Sensor
  Multiply : Gain  Gain=10^-5
  PS-Simulink Converter : nesl_utility/PS-Simulink Converter  PhysicalDomain=network_engine_domain  SubClassName=ps_output  LeftPortType=input  RightPortType=output  PseudoPeriodic=off  Frequencies=[]  Unit=inherit  AffineConversion=off
  A : PMIOPort  Side=Left
  B : PMIOPort  Port=2  Side=Left
  pressure_drop : Outport
  wires:
  PS-Simulink Converter/1 -> Multiply/1  "pa"
  Multiply/1 -> pressure_drop/1  "bar"
  connections:
  Hydraulic Pressure Sensor/LConn1 -- A/RConn1
  Hydraulic Pressure Sensor/RConn2 -- PS-Simulink Converter/LConn1
  Hydraulic Pressure Sensor/RConn1 -- B/RConn1

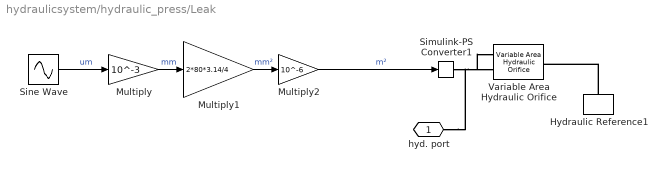
== system hydraulicsystem/hydraulic_press/Leak ==
  Hydraulic Reference1 : fl_lib/Hydraulic/Hydraulic Elements/Hydraulic Reference
  Multiply : Gain  Gain=10^-3
  Multiply1 : Gain  Gain=2*80*3.14/4
  Multiply2 : Gain  Gain=10^-6
  Simulink-PS Converter1 : nesl_utility/Simulink-PS Converter  PhysicalDomain=network_engine_domain  SubClassName=ps_input  LeftPortType=input  RightPortType=output  PseudoPeriodic=off  Frequencies=[]  NoiseDistribution=none  NoiseParameters=[]  Unit=1  AffineConversion=off  FilteringAndDerivatives=provide  SimscapeFilterOrder=1  InputFilterTimeConstant=0.001  UdotUserProvided=0
  Sine Wave : Sin  Amplitude=75  Frequency=0.001  SampleTime=0
  Variable Area Hydraulic Orifice : fl_lib/Hydraulic/Hydraulic Elements/Variable Area Hydraulic Orifice  C_d=0.1  min_area=1e-30 mm^2  lam_spec=1  B_lam=0.999  Re_cr=12  q_specify=off  q_priority=None  q=0.001 m^3/s  q_nominal_specify=off  q_nominal_unit=m^3/s  q_nominal_value=1  p_specify=off  p_priority=None  p=0 Pa  p_nominal_specify=off  p_nominal_unit=Pa  p_nominal_value=1
      settings: SourceProductBaseCode=SS  InternalSimscapePortConfiguration="{\"Bottom\":[],\"Left\":[{\"id\":\"AR\",\"label\":\"AR\",\"type\":\"input\"},{\"id\":\"A\",\"label\":\"A\",\"type\":\"foundation.hydraulic.hydraulic\"}],\"Right\":[{\"id\":\"B\",\"label\":\"B\",\"type\":\"foundation.hydraulic.hydraulic\"}],\"Top\":[]}"
  hyd. port : PMIOPort  Side=Left
  wires:
  Sine Wave/1 -> Multiply/1  "um"
  Multiply/1 -> Multiply1/1  "mm"
  Multiply2/1 -> Simulink-PS Converter1/1  "m²"
  Multiply1/1 -> Multiply2/1  "mm²"
  connections:
  Simulink-PS Converter1/RConn1 -- Variable Area Hydraulic Orifice/LConn1
  hyd. port/RConn1 -- Variable Area Hydraulic Orifice/LConn2
  Hydraulic Reference1/LConn1 -- Variable Area Hydraulic Orifice/RConn1
